simulink model "Model_Uebung_3A"  (R2021a)
settings: Solver=VariableStepAuto  StartTime=0.0  StopTime=6000  RelTol=1e-3
values from neighbouring files (symbols this model uses):
  A = [1 -1.6 0.64]    [init_uebun3_A.m]
  Atilde = [1 -1.6 0.64]    [init_uebun3_A.m]
  B = 0.15    [init_uebun3_A.m]
  B_with_delay = [0 0 0.15]    [init_uebun3_A.m]
  Btilde = 0.15    [init_uebun3_A.m]
  C = 1    [init_uebun3_A.m]
  Ctilde = [1 0 0]    [init_uebun3_A.m]
  Delta = 1    [init_uebun3_A.m]
  P0 = p0(1)*eye(3)    [init_uebun3_A.m]
  Theta0 = [0 0 0]    [init_uebun3_A.m]
libraries: cstblocks x4
settings Model: Creator=schauer  LastModifiedBy=Tomo
settings SolverCC: AlgebraicLoopSolver=TrustRegion
settings DebuggingCC: SFMachineParentedDataDiag=warning

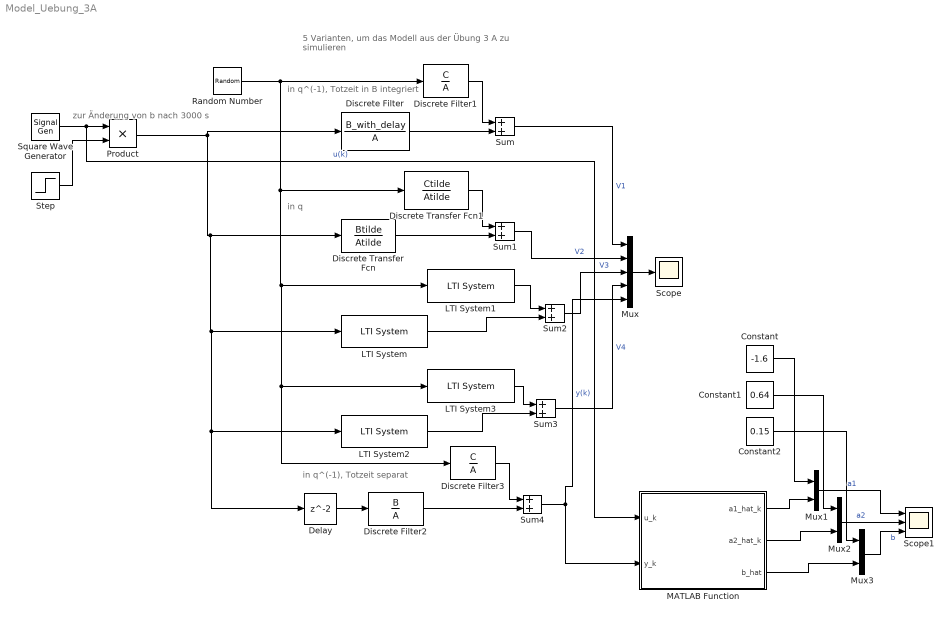
== system Model_Uebung_3A ==
  note: zur Änderung von b nach 3000 s
  note: 5 Varianten, um das Modell aus der Übung 3 A
      | zu simulieren
  note: in q^(-1), Totzeit in B integriert
  note: in q
  note: in q^(-1), Totzeit separat
  Constant : Constant  Value=-1.6
  Constant1 : Constant  Value=0.64
  Constant2 : Constant  Value=0.15
  Delay : Delay
  Discrete Transfer Fcn : DiscreteTransferFcn  Numerator=Btilde  Denominator=Atilde  SampleTime=Delta
  Discrete Transfer Fcn1 : DiscreteTransferFcn  Numerator=Ctilde  Denominator=Atilde  SampleTime=Delta
  Discrete Filter : DiscreteFilter  Numerator=B_with_delay  Denominator=A  SampleTime=Delta
  Discrete Filter1 : DiscreteFilter  Numerator=C  Denominator=A  SampleTime=Delta
  Discrete Filter2 : DiscreteFilter  Numerator=B  Denominator=A  SampleTime=Delta
  Discrete Filter3 : DiscreteFilter  Numerator=C  Denominator=A  SampleTime=Delta
  LTI System : cstblocks/LTI System  sys=G_qm1  IC=[]
  LTI System1 : cstblocks/LTI System  sys=H_qm1  IC=[]
  LTI System2 : cstblocks/LTI System  sys=G_q  IC=[]
  LTI System3 : cstblocks/LTI System  sys=H_q  IC=[]
  MATLAB Function : MATLAB Function  TreatAsAtomicUnit=on  SystemSampleTime=Delta
  Mux : Mux  Inputs=5
  Mux1 : Mux  Inputs=2
  Mux2 : Mux  Inputs=2
  Mux3 : Mux  Inputs=2
  Product : Product
  Random Number : RandomNumber  Variance=0.1^2  SampleTime=Delta
  Scope : Scope
  Scope1 : Scope  NumInputPorts=3
  Square Wave Generator : SignalGenerator  WaveForm=square  Frequency=0.01
  Step : Step  Time=3000  Before=1  After=2  SampleTime=0
  Sum{,1..4} (5 alike) : Sum
  wires:
  Discrete Filter1/1 -> Sum/1
  Discrete Filter/1 -> Sum/2
  Discrete Transfer Fcn1/1 -> Sum1/1
  Discrete Transfer Fcn/1 -> Sum1/2
  LTI System1/1 -> Sum2/1
  LTI System/1 -> Sum2/2
  LTI System3/1 -> Sum3/1
  LTI System2/1 -> Sum3/2
  Random Number/1 -> Discrete Filter3/1, LTI System3/1, LTI System1/1, Discrete Transfer Fcn1/1, Discrete Filter1/1
  Mux/1 -> Scope/1
  Sum/1 -> Mux/1  "V1"
  Sum1/1 -> Mux/2  "V2"
  Sum2/1 -> Mux/3  "V3"
  Sum3/1 -> Mux/4  "V4"
  Delay/1 -> Discrete Filter2/1
  Discrete Filter2/1 -> Sum4/2
  Discrete Filter3/1 -> Sum4/1
  Sum4/1 -> MATLAB Function/2(y_k), Mux/5  "y(k)"
  MATLAB Function/1(a1_hat_k) -> Mux1/2
  MATLAB Function/2(a2_hat_k) -> Mux2/2
  MATLAB Function/3(b_hat) -> Mux3/2
  Constant/1 -> Mux1/1
  Constant1/1 -> Mux2/1
  Constant2/1 -> Mux3/1
  Mux1/1 -> Scope1/1  "a1"
  Mux2/1 -> Scope1/2  "a2"
  Mux3/1 -> Scope1/3  "b"
  Product/1 -> Delay/1, LTI System2/1, LTI System/1, Discrete Transfer Fcn/1, Discrete Filter/1
  Square Wave Generator/1 -> MATLAB Function/1(u_k), Product/1  "u(k)"
  Step/1 -> Product/2

== matlab function Model_Uebung_3A/MATLAB Function ==
  data: u_k input; y_k input; P0 parameter; Theta0 parameter; a1_hat_k output; a2_hat_k output; b_hat output
function [a1_hat_k, a2_hat_k, b_hat] = fcn(u_k, y_k, P0, Theta0)
    d = 2;
    lambda = 0.995;
    alpha_k = 1;
    
    persistent P_k theta_hat u y step
    if isempty(P_k)
        step = 0;
        P_k = P0;
        theta_hat = Theta0';
        u = zeros(1, d);
        y = zeros(1, d);
    end
    step = step + 1;
    if step>d
        phi = [u(end-d+1) -y(end) -y(end-1)]';
        L = P_k * phi / (lambda/alpha_k + phi' * P_k * phi);
        theta_hat = theta_hat + L * (y_k - phi' * theta_hat);
        P_k = 1 / lambda * (P_k - L * phi' * P_k);
        
        u = [u(2:end) u_k];
        y = [y(2:end) y_k];
    else
        u(step) = u_k;
        y(step) = y_k;
    end
    
    b_hat = theta_hat(1);
    a1_hat_k = theta_hat(2);
    a2_hat_k = theta_hat(3);
end
